simulink model "qa_test_SDFPAdder4_A"  (Simulink 7.3)
settings: Solver=ode45  StartTime=0.0  StopTime=10.0  RelTol=1e-3
settings Model: Creator=kunal  LastModifiedBy=kunal

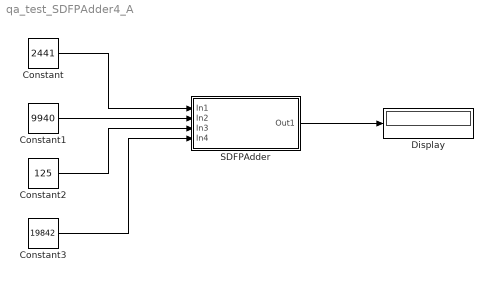
== system qa_test_SDFPAdder4_A ==
  Constant : Constant  Value=2441  OutDataTypeMode=uint32  OutDataType=fixdt(1, 16)  OutScaling=2^0  OutDataTypeStr=uint32
  Constant1 : Constant  Value=9940  OutDataTypeMode=uint32  OutDataType=fixdt(1, 16)  OutScaling=2^0  OutDataTypeStr=uint32
  Constant2 : Constant  Value=125  OutDataTypeMode=uint32  OutDataType=fixdt(1, 16)  OutScaling=2^0  OutDataTypeStr=uint32
  Constant3 : Constant  Value=19842  OutDataTypeMode=uint32  OutDataType=fixdt(1, 16)  OutScaling=2^0  OutDataTypeStr=uint32
  Display : Display
      settings: Format=hex (Stored Integer)
  SDFPAdder : Subsystem  mask{in_bitwidth=32, in_fp_position=8, out_bitwidth=32, out_fp_position=8}
      mask prompts: in_bitwidth "Input Bitwidth"; in_fp_position "Input Point Position"; out_bitwidth "Output Bitwidth"; out_fp_position "Output Point Position"
      mask Display: disp(['+\nSDFP'])
  wires:
  Constant/1 -> SDFPAdder/1(In1)
  Constant1/1 -> SDFPAdder/2(In2)
  Constant2/1 -> SDFPAdder/3(In3)
  Constant3/1 -> SDFPAdder/4(In4)
  SDFPAdder/1(Out1) -> Display/1

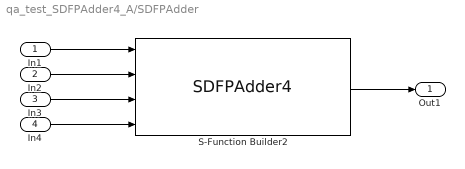
== system qa_test_SDFPAdder4_A/SDFPAdder ==
  In1 : Inport  OutDataType=fixdt(1, 16)  OutScaling=2^0
  In2 : Inport  Port=2  OutDataType=fixdt(1, 16)  OutScaling=2^0
  In3 : Inport  Port=3  OutDataType=fixdt(1, 16)  OutScaling=2^0
  In4 : Inport  Port=4  OutDataType=fixdt(1, 16)  OutScaling=2^0
  S-Function Builder2 : S-Function  InitFcn=try, set_param(gcb,'FunctionName','SDFPAdder4'), end  FunctionName=SDFPAdder4  Parameters=uint32(in_bitwidth),uint32(in_fp_position),uint32(out_bitwidth),uint32(out_fp_position)  SFunctionModules=SDFPAdder4_wrapper  WizardData=DataTag0  EnableBusSupport=off  mask(S-Function Builder){}
      mask help: The S-Function Builder block creates a wrapper C-MEX S-function from your supplied C code with multiple input ports, output ports, and a variable number of scalar, vector, or matrix parameters. The input and output ports can propagate Simulink built-in data types, fixed-point datatypes, complex, frame, 1-D, and 2-D signals. This block also supports discrete and continuous states of type real. You can optionally have the block generate a TLC file to be used with Real-Time Workshop for code generation.
      mask init:
      | val = [[.9  0.75 0.75 1 1 .9 .9 1]',[1 1 0.75 0.75 .9 .9 1 .9]'];try , sys = get_param(gcb,'SfunBuilderFcnName');if isempty(sys), sys = get_param(gcb,'FunctionName'); end,catch, sys = get_param(gcb,'FunctionName'); end
      settings: CopyFcn=set_param(gcbh,'LinkStatus','none')  PreSaveFcn=try, set_param(gcb,'FunctionName','SDFPAdder4'), end  OpenFcn=sfunctionwizard(gcbh)
      mask Display: plot(val(:,1),val(:,2)),disp(sys)port_label('input',1,'in0')port_label('input',2,'in1')port_label('input',3,'in2')port_label('input',4,'in3')port_label('output',1,'adder_out')
  Out1 : Outport  OutDataType=fixdt(1, 16)  OutScaling=2^0
  wires:
  In1/1 -> S-Function Builder2/1
  In2/1 -> S-Function Builder2/2
  In3/1 -> S-Function Builder2/3
  In4/1 -> S-Function Builder2/4
  S-Function Builder2/1 -> Out1/1
